simulink model "Book321"  (R2019b)
settings: Solver=ode4  StartTime=0.001  StopTime=3  FixedStep=0.001  RelTol=1e-3
settings Model: Creator=user  LastModifiedBy=user
settings SolverCC: AlgebraicLoopSolver=LineSearch

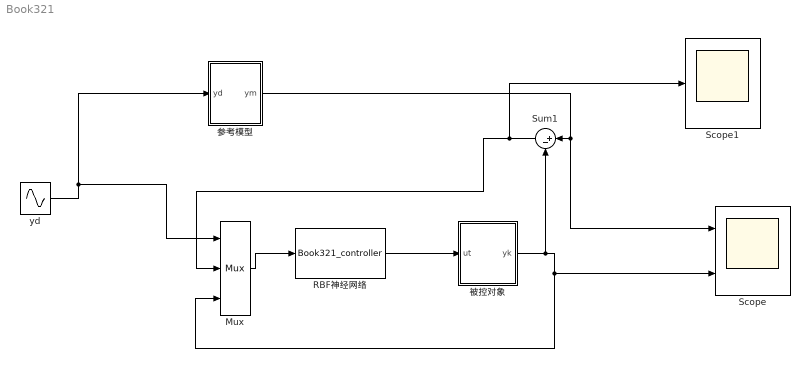
== system Book321 ==
  Mux : Mux  Inputs=3
  RBF神经网络 : S-Function  FunctionName=Book321_controller  SFunctionDeploymentMode=off  EnableBusSupport=off
  Scope : Scope  NumInputPorts=2
  Scope1 : Scope
  Sum1 : Sum  Inputs=|+-
  yd : Sin  Amplitude=0.5  Frequency=pi*2  SampleTime=0
  参考模型 : Subsystem
  被控对象 : Subsystem
  wires:
  RBF神经网络/1 -> 被控对象/1(ut)
  参考模型/1(ym) -> Scope/1, Sum1/1
  被控对象/1(yk) -> Scope/2, Mux/3, Sum1/2
  Mux/1 -> RBF神经网络/1
  yd/1 -> Mux/1, 参考模型/1(yd)
  Sum1/1 -> Scope1/1, Mux/2

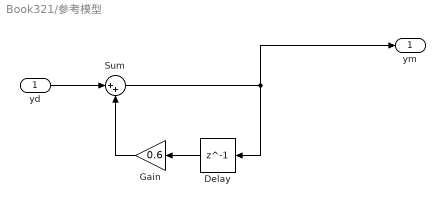
== system Book321/参考模型 ==
  yd : Inport
  Delay : Delay  DelayLength=1
  Gain : Gain  Gain=0.6
  Sum : Sum  Inputs=|++
  ym : Outport
  wires:
  yd/1 -> Sum/1
  Gain/1 -> Sum/2
  Sum/1 -> ym/1, Delay/1
  Delay/1 -> Gain/1

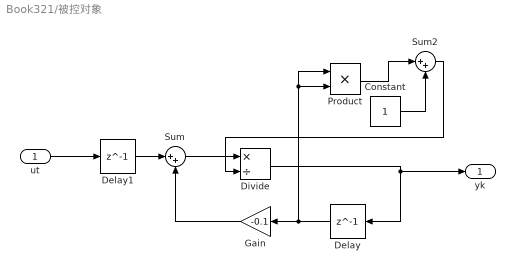
== system Book321/被控对象 ==
  ut : Inport
  Constant : Constant
  Delay : Delay  DelayLength=1
  Delay1 : Delay  DelayLength=1
  Divide : Product  Inputs=*/
  Gain : Gain  Gain=-0.1
  Product : Product
  Sum : Sum  Inputs=|++
  Sum2 : Sum  Inputs=|++
  yk : Outport
  wires:
  Delay/1 -> Product/1, Product/2, Gain/1
  Product/1 -> Sum2/1
  Divide/1 -> yk/1, Delay/1
  Sum2/1 -> Divide/2
  Sum/1 -> Divide/1
  Delay1/1 -> Sum/1
  ut/1 -> Delay1/1
  Gain/1 -> Sum/2
  Constant/1 -> Sum2/2
